simulink model "scheme"  (R2014a)
settings: Solver=ode3  StartTime=0.0  StopTime=0.005  FixedStep=1e-6  MaxStep=0.0001  MinStep=0.00001  RelTol=1e-3
settings Model: Creator=User  LastModifiedBy=trigg

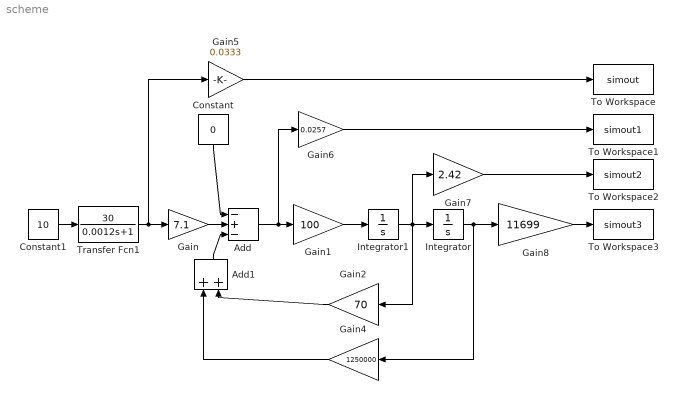
== system scheme ==
  Add : Sum  Inputs=-+-
  Add1 : Sum
  Constant : Constant  Value=0
  Constant1 : Constant  Value=10
  Gain : Gain  Gain=7.1
  Gain1 : Gain  Gain=100
  Gain2 : Gain  Gain=70
  Gain4 : Gain  Gain=1250000
  Gain5 : Gain  Gain=0.0333
  Gain6 : Gain  Gain=0.0257
  Gain7 : Gain  Gain=2.42
  Gain8 : Gain  Gain=11699
  Integrator : Integrator
  Integrator1 : Integrator
  To Workspace : ToWorkspace  VariableName=simout  SaveFormat=Timeseries  SampleTime=-1
  To Workspace1 : ToWorkspace  VariableName=simout1  SaveFormat=Timeseries  SampleTime=-1
  To Workspace2 : ToWorkspace  VariableName=simout2  SaveFormat=Timeseries  SampleTime=-1
  To Workspace3 : ToWorkspace  VariableName=simout3  SaveFormat=Timeseries  SampleTime=-1
  Transfer Fcn1 : TransferFcn  Numerator=[30]  Denominator=[0.0012 1]
  wires:
  Constant1/1 -> Transfer Fcn1/1
  Transfer Fcn1/1 -> Gain/1, Gain5/1
  Integrator1/1 -> Integrator/1, Gain2/1, Gain7/1
  Integrator/1 -> Gain8/1, Gain4/1
  Gain8/1 -> To Workspace3/1
  Gain7/1 -> To Workspace2/1
  Gain6/1 -> To Workspace1/1
  Gain5/1 -> To Workspace/1
  Gain/1 -> Add/2
  Add1/1 -> Add/3
  Add/1 -> Gain6/1, Gain1/1
  Constant/1 -> Add/1
  Gain1/1 -> Integrator1/1
  Gain2/1 -> Add1/2
  Gain4/1 -> Add1/1
